simulink model "trackTarget"  (R2017a)
settings: Solver=ode45  StartTime=tstart  StopTime=tstop  RelTol=1e-3  EnableMultiTasking=on
values from neighbouring files (symbols this model uses):
  c = 1    [run.m]
  psi0 = 50*pi/180    (= 0.872664625997)    [run.m]
  r0 = 0    [run.m]
  tsamp = 10*1    (= 10)    [run.m]
  v0 = [6.63 0]'    [run.m]
undefined symbols (not defined in the file or in its folder): msfartoystyring, WP
undefined symbols (not defined in the file): p0
libraries: simulink_extras x3, dspindex x2
settings Model: ExtModeAutoUpdateStatusClock=off  Creator=christh  LastModifiedBy=jljoberg
settings DataIOCC: LimitDataPoints=on  SaveFormat=Array  SignalLoggingSaveFormat=ModelDataLogs
settings OptimizationCC: ExpressionDepthLimit=2147483647  InitFltsAndDblsToZero=on  LifeSpan=inf
settings DebuggingCC: UnderspecifiedInitializationDetection=Classic  MergeDetectMultiDrivingBlocksExec=none  SolverPrmCheckMsg=warning  StateNameClashWarn=warning  SFUnexpectedBacktrackingDiag=warning  SFNoUnconditionalDefaultTransitionDiag=warning  SFExecutionAtInitializationDiag=none
settings HardwareCC: ProdBitPerPointer=32  ProdBitPerSizeT=32  ProdBitPerPtrDiffT=32  ProdLargestAtomicFloat=None  ProdIntDivRoundTo=Undefined  ProdEndianess=Unspecified  ProdWordSize=32  ProdHWDeviceType=32-bit Generic
settings ModelReferenceCC: PropagateSignalLabelsOutOfModel=off
settings GRTTargetCC: TargetLangStandard=C89/C90 (ANSI)  GeneratePreprocessorConditionals=Disable all  CombineOutputUpdateFcns=off  GRTInterface=on
settings ConfigComp: CovMetricSettings=dw  CovHtmlReporting=on  CovSaveCumulativeToWorkspaceVar=on  CovSaveSingleToWorkspaceVar=on  CovExternalEMLEnable=off

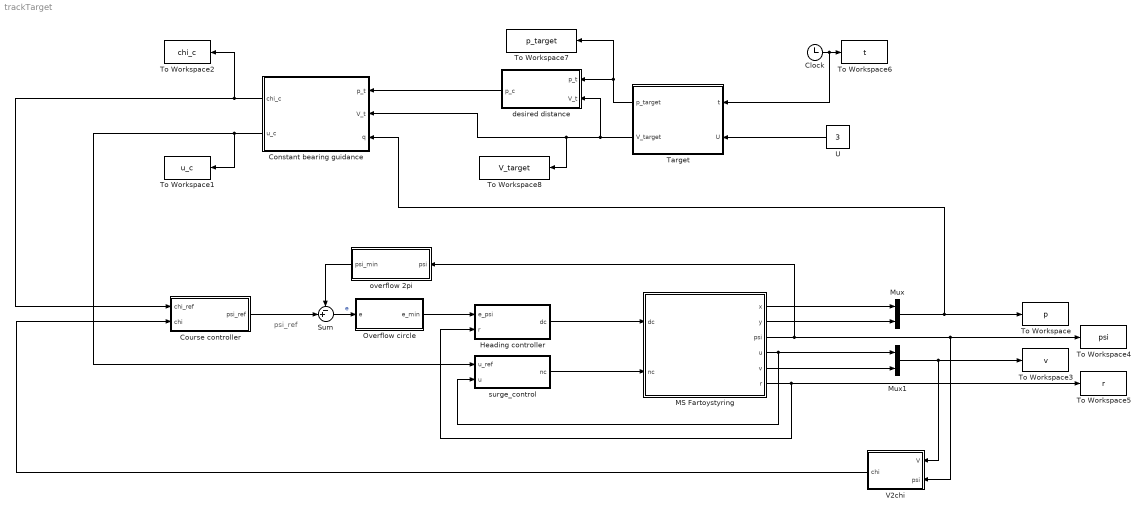
== system trackTarget ==
  note: psi_ref
  Clock : Clock
  Constant bearing guidance : MATLAB Function  TreatAsAtomicUnit=on
  Course controller : Subsystem
  Heading controller : Subsystem
  MS Fartoystyring : Subsystem  mask(MS Fartoystyring for Assignment 3 G&C){x0=p0(1), y0=p0(2), u0=v0(1), v0=v0(2), psi0=psi0, r0=r0, c=c}
      mask prompts: x0 "x(t0) (m)"; y0 "y(t0) (m)"; u0 "u(t0) (m/s)"; v0 "v(t0) (m/s)"; psi0 "psi(t0) (rad)"; r0 "r(t0) (rad/s)"; c "current (0 or 1)"
      mask help:
      | Block corresponding to Figure 1 in the assignment text. Gives the response of the ship.
      |
      | The design speed of MS Fartoystyring is u=8.23 m/s.
      |
      | Input:
      | dc: commanded rudder (rad), dmax=25*pi/180
      | nc: commanded shaft speed (rad/s), nmax=85*2*pi/60
      |
      | Output:
      | x: north pos (m)
      | y: east pos (m)
      | u: surge (m/s)
      | v: sway (m/s)
      | psi: heading (rad)
      | r: yaw (rad/s)
      mask Help: Comments, bugs and help requests can be directed to the TA. Email on course website.
  Mux : Mux  Inputs=2
  Mux1 : Mux  Inputs=2
  Overflow circle : MATLAB Function  TreatAsAtomicUnit=on
  Sum : Sum  Inputs=-+|
  Target : Subsystem
  To Workspace : ToWorkspace  VariableName=p  SampleTime=tsamp
  To Workspace1 : ToWorkspace  VariableName=u_c  SampleTime=tsamp
  To Workspace2 : ToWorkspace  VariableName=chi_c  SampleTime=tsamp
  To Workspace3 : ToWorkspace  VariableName=v  SampleTime=tsamp
  To Workspace4 : ToWorkspace  VariableName=psi  SampleTime=tsamp
  To Workspace5 : ToWorkspace  VariableName=r  SampleTime=tsamp
  To Workspace6 : ToWorkspace  VariableName=t  SampleTime=tsamp
  To Workspace7 : ToWorkspace  VariableName=p_target  SampleTime=tsamp
  To Workspace8 : ToWorkspace  VariableName=V_target  SampleTime=tsamp
  U : Constant  Value=3
  V2chi : MATLAB Function  TreatAsAtomicUnit=on
  desired distance : MATLAB Function  TreatAsAtomicUnit=on
  overflow 2pi : MATLAB Function  TreatAsAtomicUnit=on
  surge_control : Subsystem
  wires:
  Clock/1 -> Target/1(t), To Workspace6/1
  MS Fartoystyring/1(x) -> Mux/1
  MS Fartoystyring/2(y) -> Mux/2
  MS Fartoystyring/4(u) -> Mux1/1, surge_control/2(u)
  MS Fartoystyring/5(v) -> Mux1/2
  Mux1/1 -> V2chi/1(V), To Workspace3/1
  MS Fartoystyring/6(r) -> Heading controller/2(r), To Workspace5/1
  Heading controller/1(dc) -> MS Fartoystyring/1(dc)
  Mux/1 -> Constant bearing guidance/3(q), To Workspace/1
  MS Fartoystyring/3(psi) -> overflow 2pi/1(psi), To Workspace4/1, V2chi/2(psi)
  Sum/1 -> Overflow circle/1(e)  "e"
  Course controller/1(psi_ref) -> Sum/2
  V2chi/1(chi) -> Course controller/2(chi)
  surge_control/1(nc) -> MS Fartoystyring/2(nc)
  Overflow circle/1(e_min) -> Heading controller/1(e_psi)
  U/1 -> Target/2("U ")
  Target/2(V_target) -> To Workspace8/1, Constant bearing guidance/2(V_t), desired distance/2(V_t)
  Target/1(p_target) -> desired distance/1(p_t), To Workspace7/1
  Constant bearing guidance/2(u_c) -> To Workspace1/1, surge_control/1(u_ref)
  Constant bearing guidance/1(chi_c) -> Course controller/1(chi_ref), To Workspace2/1
  overflow 2pi/1(psi_min) -> Sum/1
  desired distance/1(p_c) -> Constant bearing guidance/1(p_t)

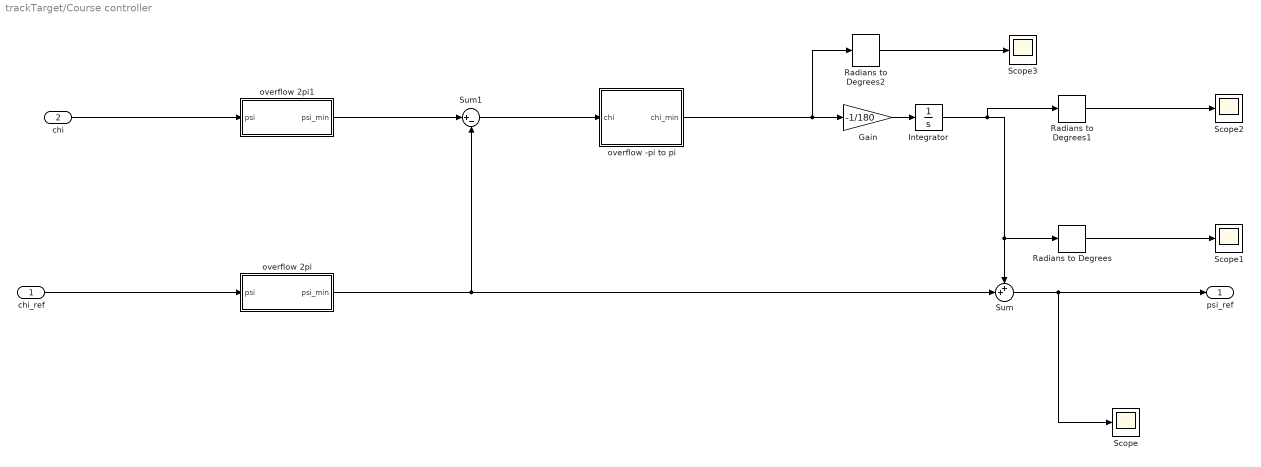
== system trackTarget/Course controller ==
  chi_ref : Inport
  chi : Inport  Port=2
  Gain : Gain  Gain=-1/180
  Integrator : Integrator  UpperSaturationLimit=90*pi/180  LowerSaturationLimit=-90*pi/180
  Radians to Degrees : simulink_extras/Transformations/Radians to Degrees
  Radians to Degrees1 : simulink_extras/Transformations/Radians to Degrees
  Radians to Degrees2 : simulink_extras/Transformations/Radians to Degrees
  Scope{,1..3} (4 alike) : Scope
  Sum : Sum  Inputs=++|
  Sum1 : Sum  Inputs=|+-
  overflow -pi to pi : MATLAB Function  TreatAsAtomicUnit=on
  overflow 2pi : MATLAB Function  TreatAsAtomicUnit=on
  overflow 2pi1 : MATLAB Function  TreatAsAtomicUnit=on
  psi_ref : Outport
  wires:
  Sum/1 -> Scope/1, psi_ref/1
  chi_ref/1 -> overflow 2pi/1(psi)
  Gain/1 -> Integrator/1
  Radians to Degrees/1 -> Scope1/1
  Sum1/1 -> overflow -pi to pi/1(chi)
  Radians to Degrees1/1 -> Scope2/1
  Integrator/1 -> Radians to Degrees1/1, Radians to Degrees/1, Sum/1
  Radians to Degrees2/1 -> Scope3/1
  chi/1 -> overflow 2pi1/1(psi)
  overflow 2pi/1(psi_min) -> Sum/2, Sum1/2
  overflow 2pi1/1(psi_min) -> Sum1/1
  overflow -pi to pi/1(chi_min) -> Radians to Degrees2/1, Gain/1

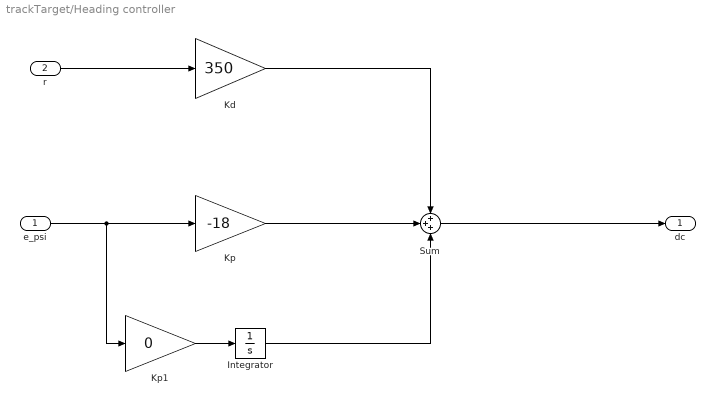
== system trackTarget/Heading controller ==
  e_psi : Inport
  r : Inport  Port=2
  Integrator : Integrator
  Kd : Gain  Gain=350
  Kp : Gain  Gain=-18
  Kp1 : Gain  Gain=0
  Sum : Sum  Inputs=+++
  dc : Outport
  wires:
  e_psi/1 -> Kp1/1, Kp/1
  Sum/1 -> dc/1
  Kp/1 -> Sum/2
  r/1 -> Kd/1
  Kd/1 -> Sum/1
  Kp1/1 -> Integrator/1
  Integrator/1 -> Sum/3

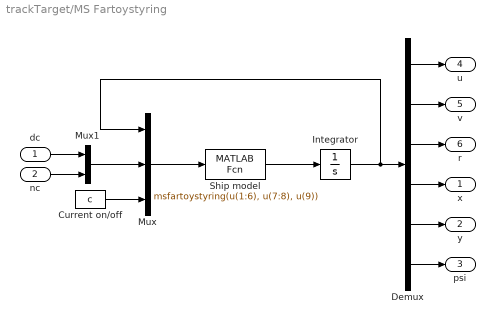
== system trackTarget/MS Fartoystyring ==
  dc : Inport
  nc : Inport  Port=2
  Current on/off : Constant  Value=c
  Demux : Demux  Outputs=6
  Integrator : Integrator  InitialCondition=[u0 v0 r0 x0 y0 psi0]'
  Mux : Mux  Inputs=3
  Mux1 : Mux  Inputs=2
  Ship model : MATLABFcn  MATLABFcn=msfartoystyring(u(1:6), u(7:8), u(9))  OutputDimensions=6
  x : Outport
  y : Outport  Port=2
  psi : Outport  Port=3
  u : Outport  Port=4
  v : Outport  Port=5
  r : Outport  Port=6
  wires:
  Integrator/1 -> Mux/1, Demux/1
  Mux1/1 -> Mux/2
  dc/1 -> Mux1/1
  nc/1 -> Mux1/2
  Demux/1 -> u/1
  Demux/2 -> v/1
  Demux/3 -> r/1
  Demux/4 -> x/1
  Demux/5 -> y/1
  Demux/6 -> psi/1
  Current on/off/1 -> Mux/3
  Ship model/1 -> Integrator/1
  Mux/1 -> Ship model/1

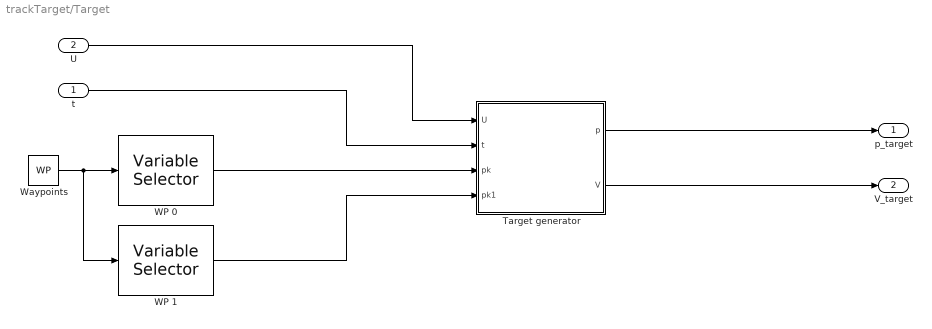
== system trackTarget/Target ==
  t : Inport
  "U " : Inport  Port=2
  Target generator : MATLAB Function  TreatAsAtomicUnit=on
  WP 0 : dspindex/Variable Selector  NumInputs=1  rowsOrCols=Columns  IdxMode=Fixed  Elements=[0]  ZerOneIdxMode=Zero-based  errmode=Clip Index  FillMode=on  FillValues=0
  WP 1 : dspindex/Variable Selector  NumInputs=1  rowsOrCols=Columns  IdxMode=Fixed  Elements=[1]  ZerOneIdxMode=Zero-based  errmode=Clip Index  FillMode=on  FillValues=0
  Waypoints : Constant  Value=WP
  p_target : Outport
  V_target : Outport  Port=2
  wires:
  Waypoints/1 -> WP 1/1, WP 0/1
  WP 1/1 -> Target generator/4(pk1)
  WP 0/1 -> Target generator/3(pk)
  t/1 -> Target generator/2(t)
  "U "/1 -> Target generator/1(U)
  Target generator/1(p) -> p_target/1
  Target generator/2(V) -> V_target/1

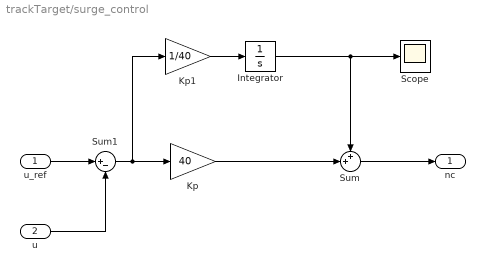
== system trackTarget/surge_control ==
  u_ref : Inport
  u : Inport  Port=2
  Integrator : Integrator  LimitOutput=on  UpperSaturationLimit=8  LowerSaturationLimit=-8
  Kp : Gain  Gain=40
  Kp1 : Gain  Gain=1/40
  Scope : Scope
  Sum : Sum  Inputs=++|
  Sum1 : Sum  Inputs=|+-
  nc : Outport
  wires:
  Sum/1 -> nc/1
  Kp/1 -> Sum/2
  Kp1/1 -> Integrator/1
  Integrator/1 -> Scope/1, Sum/1
  u/1 -> Sum1/2
  Sum1/1 -> Kp1/1, Kp/1
  u_ref/1 -> Sum1/1

== matlab function trackTarget/overflow 2pi ==
  data: psi input; psi_min output
function psi_min =  oTo2pi(psi)
psi_min = mod(psi,2*pi);

== matlab function trackTarget/Target/Target generator ==
  data: U input; p output; t input; pk input; pk1 input; V output
function [p, V]= target(U, t, pk, pk1)

s0 = 1;

pointOnLine =  @(s) pk + s*(pk1-pk);

ds = U*t/norm(pk-pk1);
p = pointOnLine(s0+ds);

V = U*[pk1(1)-pk(1); pk1(2)-pk(2)]/norm(pk1-pk);

== matlab function trackTarget/Overflow circle ==
  data: e input; e_min output
function e_min = overflow(e)
e = mod(e,2*pi);
e_min = e;
if e > pi
    e_min = e-2*pi;
end
if e < -pi
    e_min = e+2*pi;
end

== matlab function trackTarget/V2chi ==
  data: V input; chi output; psi input
function chi = V2chi(V, psi)
psi = -psi;
Rz = [cos(psi), sin(psi); -sin(psi), cos(psi)];

p_dot = Rz*V;
chi = atan2(p_dot(2), p_dot(1));

== matlab function trackTarget/Course controller/overflow -pi to pi ==
  data: chi input; chi_min output
function chi_min = overflow(chi)
chi = mod(chi, 2*pi);
chi_min = chi;
if chi > pi
    chi_min = chi-2*pi;
end
if chi < -pi
    chi_min = chi+2*pi;
end

== matlab function trackTarget/Constant bearing guidance ==
  data: p_t input; chi_c output; V_t input; q input; u_c output
function [chi_c, u_c]= get(p_t, V_t, q)

approaching_V = 20*(p_t-q)/norm(p_t-q);

if norm(p_t-q) < 1000
    approaching_V = 1/400*(p_t-q);
end


desired_V = V_t + approaching_V;

chi_c = atan2(desired_V(2), desired_V(1));
u_c = norm(desired_V);

== matlab function trackTarget/Course controller/overflow 2pi ==
  data: psi input; psi_min output
function psi_min =  oTo2pi(psi)
psi_min = mod(psi,2*pi);

== matlab function trackTarget/Course controller/overflow 2pi1 ==
  data: psi input; psi_min output
function psi_min =  oTo2pi(psi)
psi_min = mod(psi,2*pi);

== matlab function trackTarget/desired distance ==
  data: p_t input; p_c output; V_t input
function p_c = fcn(p_t, V_t)

desired_distance = 400;

p_c = p_t - desired_distance * V_t/norm(V_t);
